simulink model "finaldq1"  (R2022b)
settings: Solver=VariableStepAuto  StartTime=0.0  StopTime=1  RelTol=1e-3
libraries: spsSeriesRLCBranchLib x14, spsIGBTDiodeLib x7, spsCurrentMeasurementLib x3, spsVoltageMeasurementLib x3, simulink x2, spsAlphaBetaZerotodq0Lib x2, spsabctoAlphaBetaZeroLib x2, spsDiodeLib x1, slpidlib x1, spsThreePhaseVIMeasurementLib x1, spsThreePhaseSourceLib x1, spsdq0toabcLib x1
settings Model: SimulationMode=accelerator  Creator=91988  LastModifiedBy=AKHILA
settings SolverCC: ZeroCrossAlgorithm=Adaptive
settings DebuggingCC: IgnoredZcDiagnostic=none  UnconnectedInputMsg=warning  UnconnectedOutputMsg=warning  UnconnectedLineMsg=warning
settings ModelReferenceCC: EnableRefExpFcnMdlSchedulingChecks=on
settings RTWCC: DLArmComputeVersion=19.05

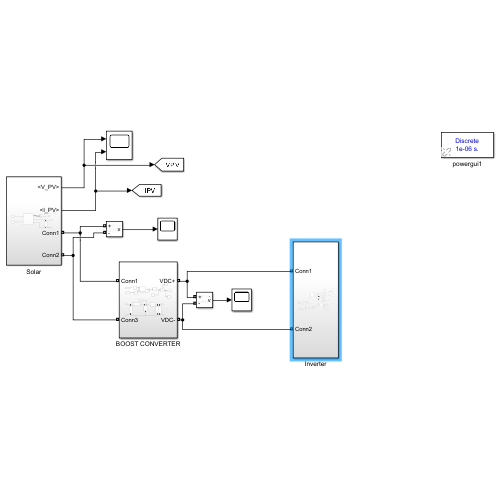
[thumbnail: Simulink's stored preview of the top-level diagram]
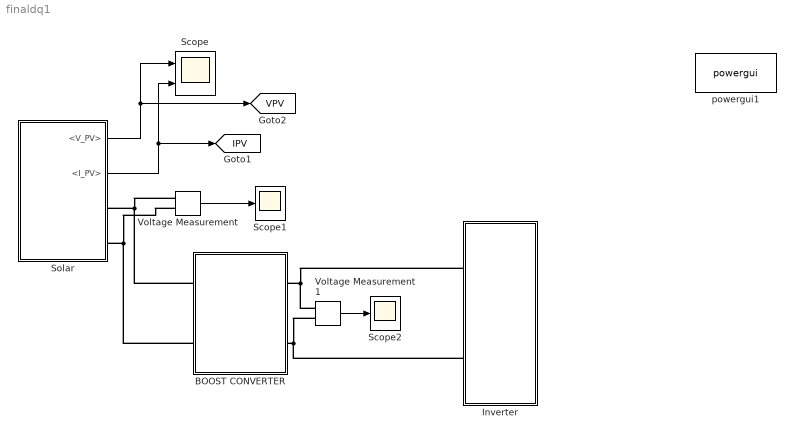
== system finaldq1 ==
  BOOST CONVERTER : Subsystem
  Inverter : Subsystem
  Scope : Scope  NumInputPorts=2
  Scope1 : Scope
  Scope2 : Scope
  Solar : Subsystem
  Voltage Measurement : spsVoltageMeasurementLib/Voltage Measurement  PhasorSimulation=off  OutputType=Complex  PSBequivalent=0
  Voltage Measurement1 : spsVoltageMeasurementLib/Voltage Measurement  PhasorSimulation=off  OutputType=Complex  PSBequivalent=0
  powergui1 : spspowerguiLib/powergui  Priority=1  SimulationMode=Discrete  SampleTime=1e-06  frequency=60  Iterations=50  frequencyindice=0  Pbase=100e6  ErrMax=1e-4  UnitsV=kV  UnitsW=MW  buscounter=0  FunctionMessages=off  echomessages=off  EnableUseOfTLC=off  CurrentSourceSwitches=off  DisableSnubberDevices=off  DisableRonSwitches=off  DisableVfSwitches=off  DisplayEquations=off  AutomaticDiscreteSolvers=off  SolverType=Tustin/Backward Euler (TBE)  Interpol=off  ExternalGateDelay=off  methode=off  Ts=100  x0status=blocks  SPID=on  SwTol=0  HookPort=off  NonlinearTolerance=1e-4  nMaxIteration=100  ContinueOnMaxIteration=off  RestoreLinks=warning  ResistiveCurrentMeasurement=off  Frange=[0:2:500]  Ylog=off  Xlog=on  ShowGrid=off  save=off  variable=ZData  structure=0  ZoomFFT=off  StartTime=0.0  cycles=1  DisplayStyle=1  fundamental=60  FreqAxis=off  MaxFrequency=1000  frequencyindicesteady=1  RmsSteady=1  display=off
  tag scope: IPV=global, VPV=global
  wires:
  Voltage Measurement/1 -> Scope1/1
  Voltage Measurement1/1 -> Scope2/1
  Solar/2(<I_PV>) -> [IPV], Scope/2
  Solar/1(<V_PV>) -> [VPV], Scope/1
  connections:
  Voltage Measurement1/LConn1 -- Inverter/LConn1 -- BOOST CONVERTER/RConn1
  Voltage Measurement1/LConn2 -- Inverter/LConn2 -- BOOST CONVERTER/RConn2
  Voltage Measurement/LConn2 -- BOOST CONVERTER/LConn2 -- Solar/RConn2
  BOOST CONVERTER/LConn1 -- Voltage Measurement/LConn1 -- Solar/RConn1

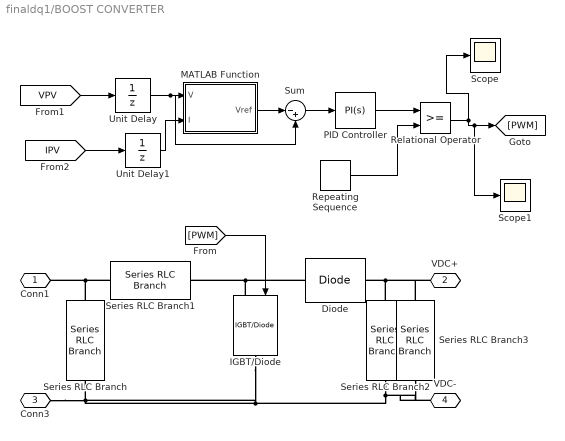
== system finaldq1/BOOST CONVERTER ==
  Diode : spsDiodeLib/Diode  Ron=0.001  Lon=0  Vf=0.8  IC=0  UseSnubber=0  Rs=500  Cs=250e-9  Measurements=off
  IGBT/Diode : spsIGBTDiodeLib/IGBT//Diode  Ron=1e-3  Rs=1e5  Cs=inf  Measurements=off
  MATLAB Function : MATLAB Function  TreatAsAtomicUnit=on
  PID Controller : slpidlib/PID Controller  Controller=PI  Form=Parallel  TimeDomain=Continuous-time  UseExternalTs=off  SampleTime=-1  IntegratorMethod=Forward Euler  FilterMethod=Forward Euler  ControllerParametersSource=internal  P=0.001  I=0.01  UseKiTs=off  D=0  N=100  UseFilter=on  TunerSelectOption=Transfer Function Based (PID Tuner App)  InitialConditionSource=internal  InitialConditionForIntegrator=0  InitialConditionForFilter=0  DifferentiatorICPrevScaledInput=0  ExternalReset=none  TrackingMode=off  Kt=1  LimitOutput=on  SatLimitsSource=internal  UpperSaturationLimit=0.95  LowerSaturationLimit=0  LinearizeAsGain=on  AntiWindupMode=none  Kb=1  LimitIntegrator=off  UpperIntegratorSaturationLimit=inf  LowerIntegratorSaturationLimit=-inf  POutMin=[]  POutMax=[]  IOutMin=[]  IOutMax=[]  DOutMin=[]  DOutMax=[]  NOutMin=[]  NOutMax=[]  SumOutMin=[]  SumOutMax=[]  SaturationOutMin=[]  SaturationOutMax=[]  PParamMin=[]  PParamMax=[]  IParamMin=[]  IParamMax=[]  DParamMin=[]  DParamMax=[]  NParamMin=[]  NParamMax=[]  KbParamMin=[]  KbParamMax=[]  KtParamMin=[]  KtParamMax=[]  KbOutMin=[]  KbOutMax=[]  KtOutMin=[]  KtOutMax=[]  IntegratorOutMin=[]  IntegratorOutMax=[]  FilterOutMin=[]  FilterOutMax=[]  SumI1OutMin=[]  SumI1OutMax=[]  SumI2OutMin=[]  SumI2OutMax=[]  SumI3OutMin=[]  SumI3OutMax=[]  SumI4OutMin=[]  SumI4OutMax=[]  SumDOutMin=[]  SumDOutMax=[]  DifferentiatorOutMin=[]  DifferentiatorOutMax=[]  FilterDiffOutCoefMin=[]  FilterDiffOutCoefMax=[]  ReciprocalOutMin=[]  ReciprocalOutMax=[]  SumDenOutMin=[]  SumDenOutMax=[]  SumNumOutMin=[]  SumNumOutMax=[]  DivideOutMin=[]  DivideOutMax=[]  UdiffTsProdOutMin=[]  UdiffTsProdOutMax=[]  NTsProdOutMin=[]  NTsProdOutMax=[]  UintegralTsProdOutMin=[]  UintegralTsProdOutMax=[]  UngainTsProdOutMin=[]  UngainTsProdOutMax=[]  ClampingZeroOutDataTypeStr=Inherit: Inherit via back propagation  ClampingZeroOutMin=[]  ClampingZeroOutMax=[]  FilterDenConstantOutDataTypeStr=Inherit: Inherit via back propagation  FilterDenConstantOutMin=[]  FilterDenConstantOutMax=[]  PCopyOutDataTypeStr=Inherit: Inherit via back propagation  PCopyOutMin=[]  PCopyOutMax=[]  NCopyOutDataTypeStr=Inherit: Inherit via back propagation  NCopyOutMin=[]  NCopyOutMax=[]  IntegratorContinuousStateAttributes=''  IntegratorStateMustResolveToSignalObject=off  IntegratorRTWStateStorageClass=Auto  FilterContinuousStateAttributes=''  FilterStateMustResolveToSignalObject=off  FilterRTWStateStorageClass=Auto  ParallelPVariant=InternalParameters  IdealPVariant=Disabled  IVariant=InternalParameters  DVariant=Disabled  IntegratorVariant=Continuous  SatVariant=Enabled  AWVariant=Passthrough  PCopyVariant=Disabled  TRVariant=Disabled  FdbkBlocksVariant=Forward  IdealPFdbkVariant=Disabled  SatFdbkVariant=Disabled  DerivativeFilterVariant=Disabled  NVariant=Disabled  NCopyVariant=Disabled_SignalSpec  FilterICVariant=Disabled  IntegratorICVariant=InternalICs  ExternalResetVariant=Disabled  TRSumVariant=Passthrough  SumFdbkVariant=Disabled  SumVariant=Sum_PI  TsampFilterVariant=InternalTs  TsampNgainVariant=Passthrough  TsampIntegralVariant=Passthrough  ExternalSaturationOutDataTypeStr=Inherit: Same as second input
  Relational Operator : RelationalOperator  OutDataTypeStr=boolean  RndMeth=Simplest  InputSameDT=off
  Repeating Sequence : simulink/Sources/Repeating Sequence  rep_seq_t=[0 0.0002]  rep_seq_y=[0 1]
  Scope : Scope
  Scope1 : Scope
  Series RLC Branch : spsSeriesRLCBranchLib/Series RLC Branch  LConnTagsString=__new0  RConnTagsString=__new0  BranchType=RC  Resistance=0.0001  Inductance=1e-3  SetiL0=off  InitialCurrent=0  Capacitance=1000e-6  Setx0=off  InitialVoltage=0  Measurements=None
  Series RLC Branch1 : spsSeriesRLCBranchLib/Series RLC Branch  LConnTagsString=__new0  RConnTagsString=__new0  BranchType=L  Resistance=1e-3  Inductance=1.45e-6  SetiL0=off  InitialCurrent=0  Capacitance=1000e-6  Setx0=off  InitialVoltage=0  Measurements=None
  Series RLC Branch2 : spsSeriesRLCBranchLib/Series RLC Branch  LConnTagsString=__new0  RConnTagsString=__new0  BranchType=C  Resistance=1e-3  Inductance=1.45e-3  SetiL0=off  InitialCurrent=0  Capacitance=3227e-6  Setx0=off  InitialVoltage=0  Measurements=None
  Series RLC Branch3 : spsSeriesRLCBranchLib/Series RLC Branch  LConnTagsString=__new0  RConnTagsString=__new0  BranchType=R  Resistance=210  Inductance=1.45e-3  SetiL0=off  InitialCurrent=0  Capacitance=3227e-6  Setx0=off  InitialVoltage=0  Measurements=None
  Sum : Sum  Inputs=|-+
  Unit Delay : UnitDelay  SampleTime=1e-06  HasFrameUpgradeWarning=on
  Unit Delay1 : UnitDelay  SampleTime=1e-06  HasFrameUpgradeWarning=on
  Conn1 : PMIOPort  Side=Left
  VDC+ : PMIOPort  Port=2  Side=Right
  Conn3 : PMIOPort  Port=3  Side=Left
  VDC- : PMIOPort  Port=4  Side=Right
  wires:
  [PWM] -> IGBT/Diode/1
  Repeating Sequence/1 -> Relational Operator/2
  [VPV] -> Unit Delay/1
  MATLAB Function/1(Vref) -> Sum/1
  PID Controller/1 -> Relational Operator/1
  [IPV] -> Unit Delay1/1
  Sum/1 -> PID Controller/1
  Relational Operator/1 -> Scope1/1, [PWM], Scope/1
  Unit Delay/1 -> Sum/2, MATLAB Function/1(V)
  Unit Delay1/1 -> MATLAB Function/2(I)
  connections:
  Conn3/RConn1 -- Series RLC Branch/RConn1 -- Series RLC Branch3/LConn1 -- VDC-/RConn1 -- Series RLC Branch2/LConn1 -- IGBT/Diode/RConn1
  Series RLC Branch/LConn1 -- Conn1/RConn1 -- Series RLC Branch1/RConn1
  IGBT/Diode/LConn1 -- Series RLC Branch1/LConn1 -- Diode/LConn1
  Series RLC Branch2/RConn1 -- Series RLC Branch3/RConn1 -- VDC+/RConn1 -- Diode/RConn1

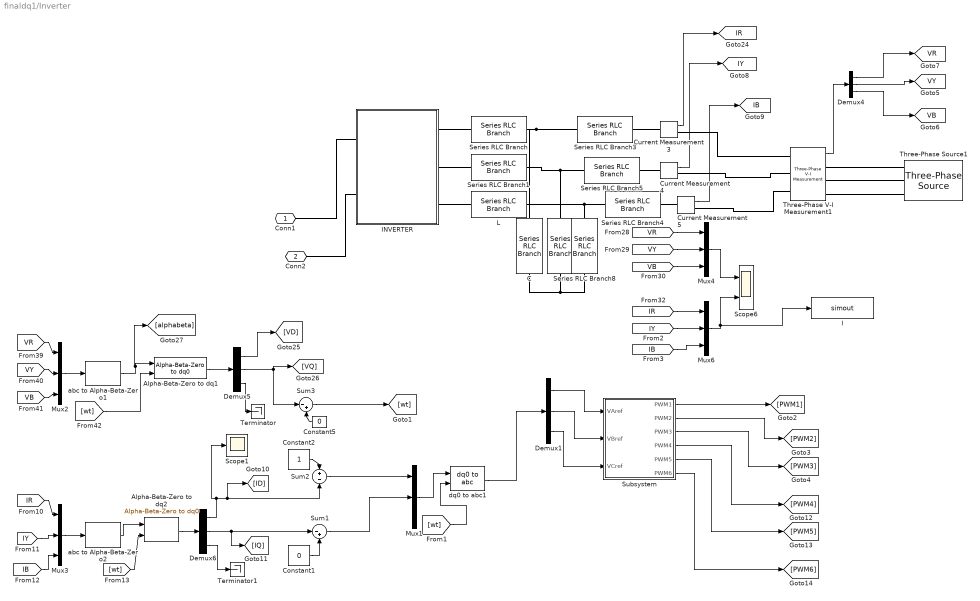
== system finaldq1/Inverter ==
  " " : spsSeriesRLCBranchLib/Series RLC Branch  LConnTagsString=__new0  RConnTagsString=__new0  BranchType=C  Resistance=1  Inductance=500e-6  SetiL0=off  InitialCurrent=0  Capacitance=1e-6  Setx0=off  InitialVoltage=0  Measurements=None
  "    C" : spsSeriesRLCBranchLib/Series RLC Branch  LConnTagsString=__new0  RConnTagsString=__new0  BranchType=C  Resistance=1  Inductance=500e-6  SetiL0=off  InitialCurrent=0  Capacitance=1e-6  Setx0=off  InitialVoltage=0  Measurements=None
  Alpha-Beta-Zero to dq1 : spsAlphaBetaZerotodq0Lib/Alpha-Beta-Zero to dq0  Alignment=90 degrees behind phase A axis
  Alpha-Beta-Zero to dq2 : spsAlphaBetaZerotodq0Lib/Alpha-Beta-Zero to dq0  Alignment=90 degrees behind phase A axis
  Constant1 : Constant  Value=0
  Constant2 : Constant
  Constant5 : Constant  Value=0
  Current Measurement3 : spsCurrentMeasurementLib/Current Measurement  PhasorSimulation=off  OutputType=Complex  PSBequivalent=0
  Current Measurement4 : spsCurrentMeasurementLib/Current Measurement  PhasorSimulation=off  OutputType=Complex  PSBequivalent=0
  Current Measurement5 : spsCurrentMeasurementLib/Current Measurement  PhasorSimulation=off  OutputType=Complex  PSBequivalent=0
  Demux{1,4..6} (4 alike) : Demux  Outputs=3
  I : ToWorkspace  VariableName=simout  SaveFormat=Timeseries  SampleTime=-1
  INVERTER : Subsystem
  L : spsSeriesRLCBranchLib/Series RLC Branch  LConnTagsString=__new0  RConnTagsString=__new0  BranchType=L  Resistance=1  Inductance=1500e-3  SetiL0=off  InitialCurrent=0  Capacitance=1e-6  Setx0=off  InitialVoltage=0  Measurements=None
  Mux{1..4,6} (5 alike) : Mux  Inputs=3
  Scope1 : Scope
  Scope6 : Scope  NumInputPorts=2
  Series RLC Branch{,1,3..5} (5 alike) : spsSeriesRLCBranchLib/Series RLC Branch  LConnTagsString=__new0  RConnTagsString=__new0  BranchType=L  Resistance=1  Inductance=1500e-3  SetiL0=off  InitialCurrent=0  Capacitance=1e-6  Setx0=off  InitialVoltage=0  Measurements=None
  Series RLC Branch8 : spsSeriesRLCBranchLib/Series RLC Branch  LConnTagsString=__new0  RConnTagsString=__new0  BranchType=C  Resistance=1  Inductance=500e-6  SetiL0=off  InitialCurrent=0  Capacitance=1e-6  Setx0=off  InitialVoltage=0  Measurements=None
  Subsystem : Subsystem
  Sum1 : Sum  Inputs=|-+
  Sum2 : Sum  Inputs=+-
  Sum3 : Sum  Inputs=|-+
  Terminator : Terminator
  Terminator1 : Terminator
  Three-Phase V-I Measurement1 : spsThreePhaseVIMeasurementLib/Three-Phase V-I Measurement  VoltageMeasurement=phase-to-phase  SetLabelV=off  LabelV=Vabc  Vpu=off  VpuLL=off  CurrentMeasurement=no  SetLabelI=off  LabelI=Iabc  Ipu=off  Pbase=100e6  Vbase=500e3  OutputType=Complex  PhasorSimulation=off  PSBequivalent=0
  Three-Phase Source1 : spsThreePhaseSourceLib/Three-Phase Source  InternalConnection=Y  VoltagePhases=off  Voltage=415  PhaseAngle=0  Voltage_phases=[25e3 25e3 25e3]/sqrt(3)  PhaseAngles_phases=[0 -120 +120]  Frequency=50  NonIdealSource=on  SpecifyImpedance=off  Resistance=0.001e-3  Inductance=0.001e-9  ShortCircuitLevel=100e6  BaseVoltage=415  XRratio=7  BusType=swing  Pref=10e3  Qref=0  Prefabc=[10e3, 10e3, 10e3]  Qrefabc=[0, 0, 0]  Qmin=-inf  Qmax=inf
  abc to Alpha-Beta-Zero1 : spsabctoAlphaBetaZeroLib/abc to Alpha-Beta-Zero
  abc to Alpha-Beta-Zero2 : spsabctoAlphaBetaZeroLib/abc to Alpha-Beta-Zero
  dq0 to abc1 : spsdq0toabcLib/dq0 to abc  Alignment=90 degrees behind phase A axis
  Conn1 : PMIOPort  Side=Left
  Conn2 : PMIOPort  Port=2  Side=Left
  tag scope: IB=global, IR=global, IY=global, VB=global, VR=global, VY=global
  wires:
  [VY] -> Mux2/2
  abc to Alpha-Beta-Zero1/1 -> [alphabeta], Alpha-Beta-Zero to dq1/1
  Demux6/2 -> Sum1/1, [IQ]
  Mux3/1 -> abc to Alpha-Beta-Zero2/1
  [VR] -> Mux2/1
  Demux5/2 -> [VQ], Sum3/1
  [VB] -> Mux2/3
  [IY] -> Mux3/2
  Mux2/1 -> abc to Alpha-Beta-Zero1/1
  Demux5/1 -> [VD]
  Demux6/1 -> Sum2/2, [ID], Scope1/1
  [wt] -> Alpha-Beta-Zero to dq2/2
  abc to Alpha-Beta-Zero2/1 -> Alpha-Beta-Zero to dq2/1
  [IB] -> Mux3/3
  Alpha-Beta-Zero to dq2/1 -> Demux6/1
  [wt] -> Alpha-Beta-Zero to dq1/2
  [IR] -> Mux3/1
  Alpha-Beta-Zero to dq1/1 -> Demux5/1
  Constant5/1 -> Sum3/2
  Constant1/1 -> Sum1/2
  Mux1/1 -> dq0 to abc1/1
  [wt] -> dq0 to abc1/2
  Current Measurement5/1 -> [IB]
  Demux4/1 -> [VR]
  Three-Phase V-I Measurement1/1 -> Demux4/1
  Demux4/3 -> [VB]
  Demux4/2 -> [VY]
  [IR] -> Mux6/1
  [VR] -> Mux4/1
  [VB] -> Mux4/3
  Mux4/1 -> Scope6/1
  [VY] -> Mux4/2
  Mux6/1 -> I/1, Scope6/2
  Current Measurement4/1 -> [IY]
  Constant2/1 -> Sum2/1
  dq0 to abc1/1 -> Demux1/1
  Subsystem/1(PWM1) -> [PWM1]
  Subsystem/2(PWM2) -> [PWM2]
  Subsystem/3(PWM3) -> [PWM3]
  Subsystem/4(PWM4) -> [PWM4]
  Subsystem/5(PWM5) -> [PWM5]
  Subsystem/6(PWM6) -> [PWM6]
  Demux1/1 -> Subsystem/1(VAref)
  Demux1/2 -> Subsystem/2(VBref)
  Demux1/3 -> Subsystem/3(VCref)
  [IY] -> Mux6/2
  [IB] -> Mux6/3
  Demux5/3 -> Terminator/1
  Demux6/3 -> Terminator1/1
  Current Measurement3/1 -> [IR]
  Sum3/1 -> [wt]
  Sum2/1 -> Mux1/1
  Sum1/1 -> Mux1/2
  connections:
  Series RLC Branch8/LConn1 -- L/RConn1 -- Series RLC Branch4/LConn1
  " "/LConn1 -- Series RLC Branch5/LConn1 -- Series RLC Branch1/RConn1
  "    C"/LConn1 -- Series RLC Branch/RConn1 -- Series RLC Branch3/LConn1
  "    C"/RConn1 -- Series RLC Branch8/RConn1 -- " "/RConn1
  INVERTER/RConn2 -- Series RLC Branch1/LConn1
  Current Measurement3/RConn1 -- Three-Phase V-I Measurement1/LConn1
  Current Measurement5/LConn1 -- Series RLC Branch4/RConn1
  Current Measurement5/RConn1 -- Three-Phase V-I Measurement1/LConn3
  Current Measurement4/RConn1 -- Three-Phase V-I Measurement1/LConn2
  INVERTER/RConn3 -- L/LConn1
  Series RLC Branch5/RConn1 -- Current Measurement4/LConn1
  Three-Phase V-I Measurement1/RConn3 -- Three-Phase Source1/RConn1
  Three-Phase V-I Measurement1/RConn1 -- Three-Phase Source1/RConn3
  Current Measurement3/LConn1 -- Series RLC Branch3/RConn1
  INVERTER/RConn1 -- Series RLC Branch/LConn1
  Three-Phase V-I Measurement1/RConn2 -- Three-Phase Source1/RConn2
  Conn1/RConn1 -- INVERTER/LConn1
  Conn2/RConn1 -- INVERTER/LConn2

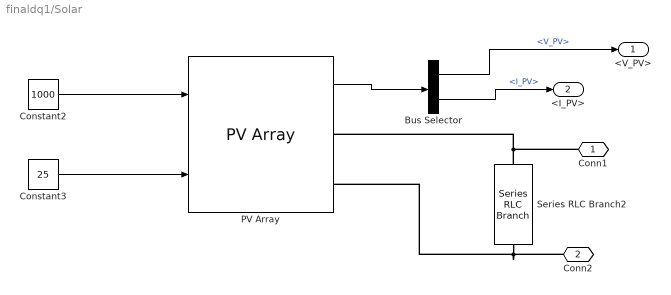
== system finaldq1/Solar ==
  Bus Selector : BusSelector  OutputSignals=V_PV,I_PV
  Constant2 : Constant  Value=1000
  Constant3 : Constant  Value=25
  PV Array : spsPVArrayLib/PV Array  Npar=1  Nser=10  PlotType=array @ 25 deg.C & specified irradiances  S_vec="[ 1000  500  100 ]"  Temp_C_vec="[ 45 25  ]"  ModuleName=User-defined  PlotWhenSelected=off  Pm=200.112  Ncell=54  Voc=32.9  Isc=8.21  Vm=26.4  Im=7.58  beta_Voc_pc=-0.36099  alpha_Isc_pc=0.102  beta_Voc=-0.11877  alpha_Isc=0.0083742  IL=8.2311  I0=3.0465e-10  nI=0.98858  Rsh=126.9934  Rs=0.32653  RobustModel=off  RobustCellTemperature=313.3991  BAL=on  Tc=1e-6  Tfilter=5e-5
  Series RLC Branch2 : spsSeriesRLCBranchLib/Series RLC Branch  LConnTagsString=__new0  RConnTagsString=__new0  BranchType=C  Resistance=34.8  Inductance=1e-3  SetiL0=off  InitialCurrent=0  Capacitance=320e-6  Setx0=off  InitialVoltage=0  Measurements=None
  Conn1 : PMIOPort  Side=Right
  Conn2 : PMIOPort  Port=2  Side=Right
  <V_PV> : Outport
  <I_PV> : Outport  Port=2
  wires:
  Bus Selector/1 -> <V_PV>/1  "<V_PV>"
  Bus Selector/2 -> <I_PV>/1  "<I_PV>"
  PV Array/1 -> Bus Selector/1
  Constant2/1 -> PV Array/1
  Constant3/1 -> PV Array/2
  connections:
  PV Array/RConn1 -- Conn1/RConn1 -- Series RLC Branch2/LConn1
  PV Array/RConn2 -- Conn2/RConn1 -- Series RLC Branch2/RConn1

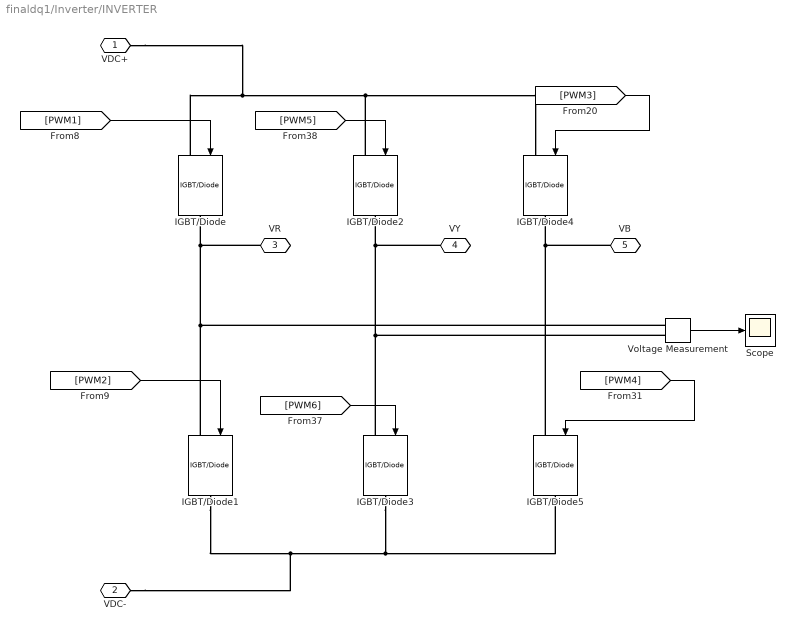
== system finaldq1/Inverter/INVERTER ==
  IGBT/Diode{,1..5} (6 alike) : spsIGBTDiodeLib/IGBT//Diode  Ron=1e-3  Rs=1e5  Cs=inf  Measurements=off
  Scope : Scope
  Voltage Measurement : spsVoltageMeasurementLib/Voltage Measurement  PhasorSimulation=off  OutputType=Complex  PSBequivalent=0
  VDC+ : PMIOPort  Side=Left
  VDC- : PMIOPort  Port=2  Side=Left
  VR : PMIOPort  Port=3  Side=Right
  VY : PMIOPort  Port=4  Side=Right
  VB : PMIOPort  Port=5  Side=Right
  wires:
  [PWM2] -> IGBT/Diode1/1
  [PWM1] -> IGBT/Diode/1
  Voltage Measurement/1 -> Scope/1
  [PWM3] -> IGBT/Diode4/1
  [PWM4] -> IGBT/Diode5/1
  [PWM5] -> IGBT/Diode2/1
  [PWM6] -> IGBT/Diode3/1
  connections:
  IGBT/Diode1/LConn1 -- VR/RConn1 -- IGBT/Diode/RConn1 -- Voltage Measurement/LConn1
  IGBT/Diode5/LConn1 -- VB/RConn1 -- IGBT/Diode4/RConn1
  IGBT/Diode/LConn1 -- VDC+/RConn1 -- IGBT/Diode2/LConn1 -- IGBT/Diode4/LConn1
  IGBT/Diode3/LConn1 -- Voltage Measurement/LConn2 -- VY/RConn1 -- IGBT/Diode2/RConn1
  IGBT/Diode1/RConn1 -- VDC-/RConn1 -- IGBT/Diode3/RConn1 -- IGBT/Diode5/RConn1

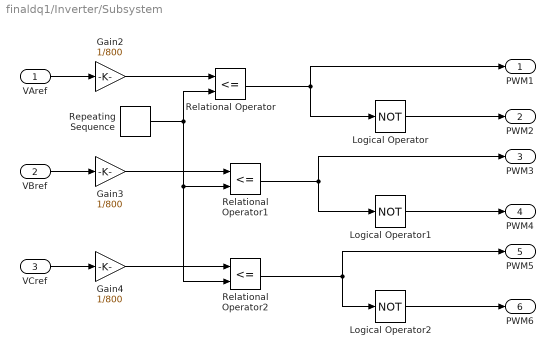
== system finaldq1/Inverter/Subsystem ==
  VAref : Inport
  VBref : Inport  Port=2
  VCref : Inport  Port=3
  Gain2 : Gain  Gain=1/800
  Gain3 : Gain  Gain=1/800
  Gain4 : Gain  Gain=1/800
  Logical Operator : Logic  Operator=NOT  AllPortsSameDT=off  OutDataTypeStr=boolean
  Logical Operator1 : Logic  Operator=NOT  AllPortsSameDT=off  OutDataTypeStr=boolean
  Logical Operator2 : Logic  Operator=NOT  AllPortsSameDT=off  OutDataTypeStr=boolean
  Relational Operator : RelationalOperator  Operator=<=  OutDataTypeStr=boolean  RndMeth=Simplest  InputSameDT=off
  Relational Operator1 : RelationalOperator  Operator=<=  OutDataTypeStr=boolean  RndMeth=Simplest  InputSameDT=off
  Relational Operator2 : RelationalOperator  Operator=<=  OutDataTypeStr=boolean  RndMeth=Simplest  InputSameDT=off
  Repeating Sequence : simulink/Sources/Repeating Sequence  rep_seq_t=[0 0.00005 0.0001]  rep_seq_y=[-1 1 -1]
  PWM1 : Outport
  PWM2 : Outport  Port=2
  PWM3 : Outport  Port=3
  PWM4 : Outport  Port=4
  PWM5 : Outport  Port=5
  PWM6 : Outport  Port=6
  wires:
  Gain2/1 -> Relational Operator/1
  VAref/1 -> Gain2/1
  Gain4/1 -> Relational Operator2/1
  VBref/1 -> Gain3/1
  Relational Operator1/1 -> PWM3/1, Logical Operator1/1
  Gain3/1 -> Relational Operator1/1
  Logical Operator/1 -> PWM2/1
  Logical Operator2/1 -> PWM6/1
  Relational Operator2/1 -> PWM5/1, Logical Operator2/1
  VCref/1 -> Gain4/1
  Repeating Sequence/1 -> Relational Operator2/2, Relational Operator1/2, Relational Operator/2
  Relational Operator/1 -> PWM1/1, Logical Operator/1
  Logical Operator1/1 -> PWM4/1

== matlab function finaldq1/BOOST CONVERTER/MATLAB Function ==
  settings: updateMethod=DISCRETE
  data: V input; Vref output; I input
function Vref = RefGen(V,I)

Vrefmax = 363;
Vrefmin = 0;
Vrefinit = 300;
deltaVref = 1;
persistent Vold Pold Vrefold;

dataType = 'double';

if isempty(Vold)
    Vold = 0;
    Pold = 0;
    Vrefold = Vrefinit;
end

P = V*I;
dV = V - Vold;
dP = P - Pold;
 
if dP ~= 0
    if dP<0
        if dV<0
            Vref = Vrefold + deltaVref;
        else
            Vref = Vrefold - deltaVref;
        end
    else
        if dV<0
            Vref = Vrefold - deltaVref;
        else
            Vref = Vrefold + deltaVref;
        end
    end
else
    Vref = Vrefold;
end

if Vref >= Vrefmax | Vref <= Vrefmin
    Vref = Vrefold;
end

Vrefold = Vref;
Vold = V;
Pold = P;
